simulink model "board_virgin_lab1"  (R2015a)
settings: Solver=ode3  StartTime=0.0  StopTime=inf  FixedStep=0.001  RelTol=1e-3
libraries: PoliArd x14, simulink x2
settings Model: ExtModeTrigDuration=2  Creator=User  LastModifiedBy=user
settings OptimizationCC: OptimizeModelRefInitCode=on  LifeSpan=1
settings DebuggingCC: UnderspecifiedInitializationDetection=Classic  MergeDetectMultiDrivingBlocksExec=none
settings HardwareCC: ProdLargestAtomicInteger=Long  ProdLargestAtomicFloat=Double  ProdEndianess=LittleEndian  ProdHWDeviceType=ARM Compatible->ARM Cortex
settings RTWCC: SystemTargetFile=realtime.tlc  GenerateMakefile=off  TemplateMakefile=realtime.tmf  Description=Run on Target Hardware  RTWVerbose=off
settings ERTTargetCC: CombineOutputUpdateFcns=off  ExtModeTransport=3  ExtModeMexFile=ext_serial_win32_comm_rtt  ExtModeMexArgs=0 1 9600  InlinedParameterPlacement=Hierarchical  ERTSrcFileBannerTemplate=realtime_code_template.cgt  ERTHdrFileBannerTemplate=realtime_code_template.cgt  ERTDataSrcFileTemplate=realtime_code_template.cgt  ERTDataHdrFileTemplate=realtime_code_template.cgt  ERTCustomFileTemplate=realtime_file_process.tlc

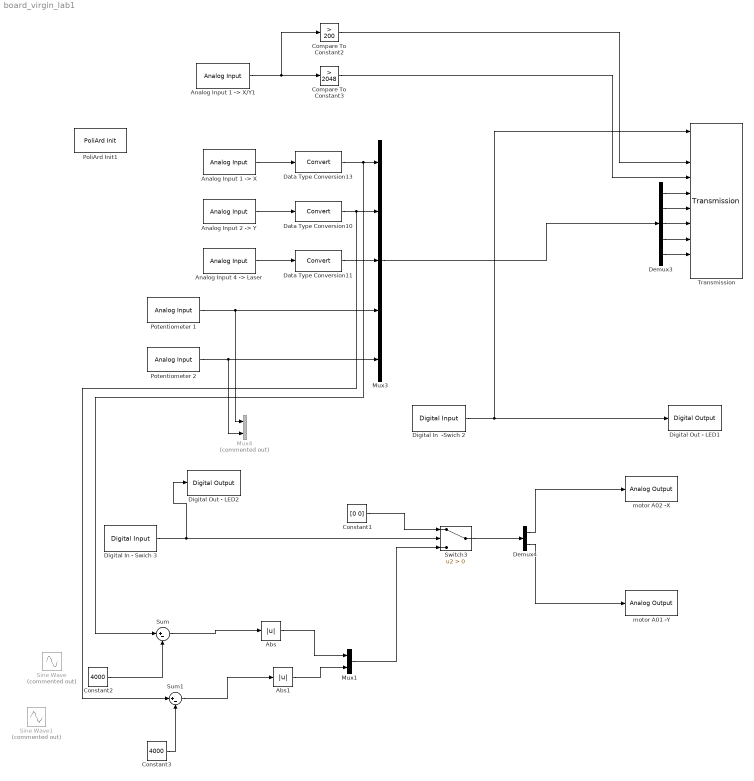
== system board_virgin_lab1 ==
  Abs : Abs
  Abs1 : Abs
  "Analog Input 1 -> X" : PoliArd/Analog Input  AIpin_mask=1  AIsample=-1
  "Analog Input 1 -> X/Y1" : PoliArd/Analog Input  AIpin_mask=7  AIsample=-1
  "Analog Input 2 -> Y" : PoliArd/Analog Input  AIpin_mask=2  AIsample=-1
  "Analog Input 4 -> Laser" : PoliArd/Analog Input  AIpin_mask=4  AIsample=-1
  Compare To Constant2 : simulink/Logic and Bit Operations/Compare To Constant  relop=>  const=200  OutDataTypeStr=boolean
  Compare To Constant3 : simulink/Logic and Bit Operations/Compare To Constant  relop=>  const=2048  OutDataTypeStr=boolean
  Constant1 : Constant  Value=[0 0]
  Constant2 : Constant  Value=4000
  Constant3 : Constant  Value=4000
  Data Type Conversion10 : DataTypeConversion
  Data Type Conversion11 : DataTypeConversion
  Data Type Conversion13 : DataTypeConversion
  Demux3 : Demux  Outputs=5
  Demux4 : Demux  Outputs=2
  Digital In  -Swich 2 : PoliArd/Digital Input  DI_pin=2  DIsample=-1
  Digital In - Swich 3 : PoliArd/Digital Input  DI_pin=3  DIsample=-1
  Digital Out - LED1 : PoliArd/Digital Output  DO_pin=1
  Digital Out - LED2 : PoliArd/Digital Output  DO_pin=2
  Mux1 : Mux  Inputs=2
  Mux3 : Mux  Inputs=5
  Mux4 : Mux  Commented=on  Inputs=2
  PoliArd Init1 : PoliArd/PoliArd Init
  Potentiometer 1 : PoliArd/Analog Input  AIpin_mask=8  AIsample=-1
  Potentiometer 2 : PoliArd/Analog Input  AIpin_mask=9  AIsample=-1
  Sine Wave : Sin  Commented=on  Amplitude=200  Bias=2000  Frequency=2 * 3.14  SampleTime=0
  Sine Wave1 : Sin  Commented=on  Amplitude=200  Bias=2000  Frequency=2 * 3.14  Phase=pi/2  SampleTime=0
  Sum : Sum  Inputs=|+-
  Sum1 : Sum  Inputs=|+-
  Switch3 : Switch  Criteria=u2 > Threshold
  Transmission : PoliArd/Transmission  sample_freq=100  sig_to_send=6
  motor A01 -Y : PoliArd/Analog Output  DAC_pin_mask=2
  motor A02 -X : PoliArd/Analog Output  DAC_pin_mask=1
  wires:
  "Analog Input 1 -> X"/1 -> Data Type Conversion13/1
  "Analog Input 2 -> Y"/1 -> Data Type Conversion10/1
  "Analog Input 4 -> Laser"/1 -> Data Type Conversion11/1
  Potentiometer 1/1 -> Mux3/4, Mux4/1
  Potentiometer 2/1 -> Mux3/5, Mux4/2
  Data Type Conversion13/1 -> Sum/1, Mux3/1
  Data Type Conversion10/1 -> Sum1/1, Mux3/2
  Data Type Conversion11/1 -> Mux3/3
  Digital In  -Swich 2/1 -> Transmission/1, Digital Out - LED1/1
  "Analog Input 1 -> X/Y1"/1 -> Compare To Constant3/1, Compare To Constant2/1
  Compare To Constant2/1 -> Transmission/3
  Compare To Constant3/1 -> Transmission/4
  Demux3/1 -> Transmission/5
  Demux3/2 -> Transmission/6
  Demux3/3 -> Transmission/7
  Demux3/4 -> Transmission/8
  Demux3/5 -> Transmission/9
  Mux3/1 -> Demux3/1
  Digital In - Swich 3/1 -> Digital Out - LED2/1, Switch3/2
  Constant1/1 -> Switch3/1
  Demux4/2 -> motor A01 -Y/1
  Demux4/1 -> motor A02 -X/1
  Switch3/1 -> Demux4/1
  Mux1/1 -> Switch3/3
  Constant2/1 -> Sum/2
  Constant3/1 -> Sum1/2
  Sum/1 -> Abs/1
  Abs/1 -> Mux1/1
  Sum1/1 -> Abs1/1
  Abs1/1 -> Mux1/2
